simulink model "CANcommunicationmodule"  (R2024a)
settings: Solver=VariableStepAuto  StartTime=0.0  StopTime=10.0  RelTol=1e-3
undefined symbols (not defined in the file or in its folder): canChannel
libraries: canlib x4, canmsglib x3
settings Model: DataDictionary=BMS_System_dict1.sldd  Creator=hirah  LastModifiedBy=hirah

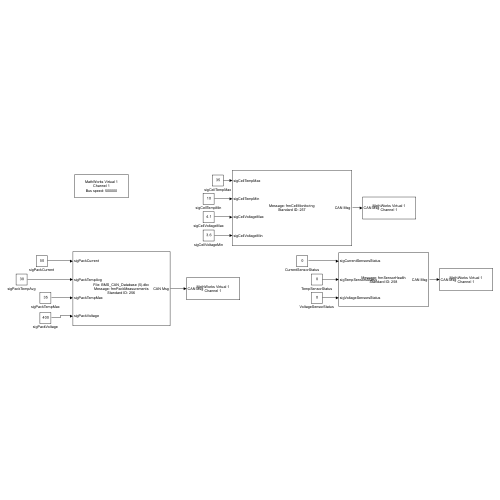
[thumbnail: Simulink's stored preview of the top-level diagram]
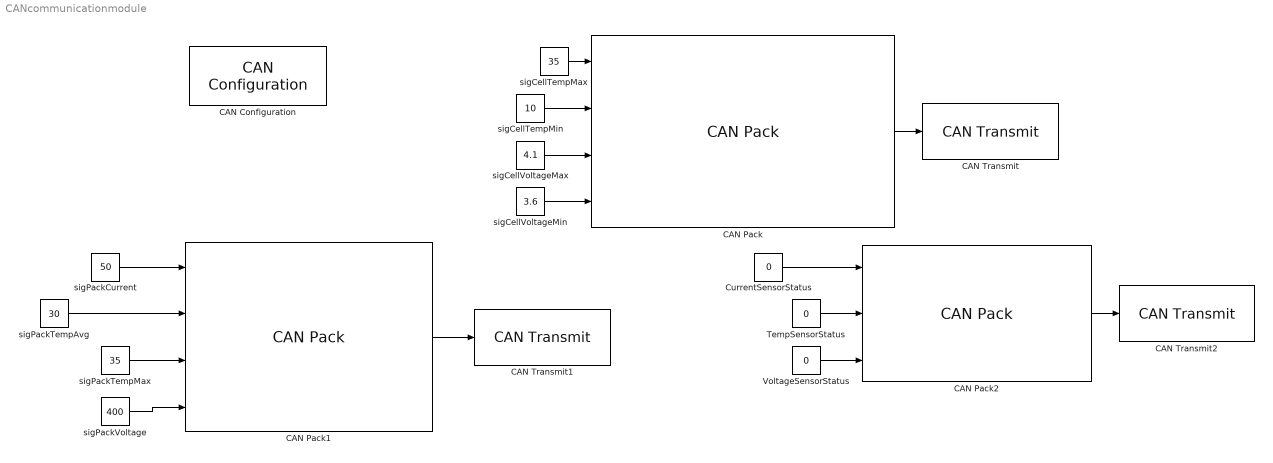
== system CANcommunicationmodule ==
  CAN Configuration : canlib/CAN Configuration  BlockHandle=788.0009  Device=MathWorks Virtual 1 (Channel 1)  DeviceMenu=MathWorks Virtual 1 (Channel 1)  ObjConstructor=canChannel('MathWorks', 'Virtual 1', 1)  BusSpeed=500000  EnableBitParameters=off  AckMode=Normal
  CAN Pack : canmsglib/CAN Pack  CANdbFile=C:\Users\hirah\Downloads\BMS_CAN_Database (5).dbc  MsgList=frmCellMonitoring  MsgName=frmCellMonitoring  MsgIDType=Standard (11-bit identifier)  MsgIdentifier=257  MsgLength=6  Remote=off  ApplyMinMax=off  BusOutput=off  SignalInfo={ 'sigCellTempMax', '32', '8', 'LE', 'unsigned', 'Standard', '0', '1', '-40', '-40', '150'; 'sigCellTempMin', '40', '8', 'LE', 'unsigned', 'Standard', '0', '1', '-40', '-40', '150'; 'sigCellVoltageMax', '0', '16', 'LE', 'unsigned', 'Standard', '0', '0.001', '0', '0', '5'; 'sigCellVoltageMin', '16', '16', 'LE', 'unsigned', 'Standard', '0', '0.001', '0', '0', '5' }
      settings: LibrarySourceBlock=canlib/CAN Pack  DataFormat=manually specified signals
  CAN Pack1 : canmsglib/CAN Pack  CANdbFile=C:\Users\hirah\Downloads\BMS_CAN_Database (5).dbc  MsgList=frmPackMeasurements  MsgName=frmPackMeasurements  MsgIDType=Standard (11-bit identifier)  MsgIdentifier=256  MsgLength=6  Remote=off  ApplyMinMax=off  BusOutput=off  SignalInfo={'sigPackCurrent','16','16','LE','signed','Standard','0','0.1','0','-400','400';'sigPackTempAvg','32','8','LE','unsigned','Standard','0','1','-40','-40','150';'sigPackTempMax','40','8','LE','unsigned','Standard','0','1','-40','-40','150';'sigPackVoltage','0','16','LE','unsigned','Standard','0','0.1','0','0','1000'}
      settings: LibrarySourceBlock=canlib/CAN Pack  DataFormat=CANdb specified signals
  CAN Pack2 : canmsglib/CAN Pack  CANdbFile=C:\Users\hirah\Downloads\BMS_CAN_Database (5).dbc  MsgList=frmSensorHealth  MsgName=frmSensorHealth  MsgIDType=Standard (11-bit identifier)  MsgIdentifier=258  MsgLength=3  Remote=off  ApplyMinMax=off  BusOutput=off  SignalInfo={ 'sigCurrentSensorsStatus', '8', '8', 'LE', 'unsigned', 'Standard', '0', '1', '0', '0', '3'; 'sigTempSensorsStatus', '16', '8', 'LE', 'unsigned', 'Standard', '0', '1', '0', '0', '3'; 'sigVoltageSensorsStatus', '0', '8', 'LE', 'unsigned', 'Standard', '0', '1', '0', '0', '3' }
      settings: LibrarySourceBlock=canlib/CAN Pack  DataFormat=manually specified signals
  CAN Transmit : canlib/CAN Transmit  BlockHandle=806.0001  Device=MathWorks Virtual 1 (Channel 1)  DeviceMenu=MathWorks Virtual 1 (Channel 1)  ObjConstructor=canChannel('MathWorks', 'Virtual 1', 1)  EnableEventTransmit=off  EnablePeriodicTransmit=off  MessagePeriod=1.000
  CAN Transmit1 : canlib/CAN Transmit  BlockHandle=808.0001  Device=MathWorks Virtual 1 (Channel 1)  DeviceMenu=MathWorks Virtual 1 (Channel 1)  ObjConstructor=canChannel('MathWorks', 'Virtual 1', 1)  EnableEventTransmit=off  EnablePeriodicTransmit=off  MessagePeriod=1.000
  CAN Transmit2 : canlib/CAN Transmit  BlockHandle=810.0001  Device=MathWorks Virtual 1 (Channel 1)  DeviceMenu=MathWorks Virtual 1 (Channel 1)  ObjConstructor=canChannel('MathWorks', 'Virtual 1', 1)  EnableEventTransmit=off  EnablePeriodicTransmit=off  MessagePeriod=1.000
  CurrentSensorStatus : Constant  Value=0  OutDataTypeStr=uint8
  TempSensorStatus : Constant  Value=0  OutDataTypeStr=uint8
  VoltageSensorStatus : Constant  Value=0  OutDataTypeStr=uint8
  sigCellTempMax : Constant  Value=35  OutDataTypeStr=int8
  sigCellTempMin : Constant  Value=10  OutDataTypeStr=int8
  sigCellVoltageMax : Constant  Value=4.1  OutDataTypeStr=double
  sigCellVoltageMin : Constant  Value=3.6  OutDataTypeStr=double
  sigPackCurrent : Constant  Value=50  OutDataTypeStr=double
  sigPackTempAvg : Constant  Value=30  OutDataTypeStr=double
  sigPackTempMax : Constant  Value=35  OutDataTypeStr=double
  sigPackVoltage : Constant  Value=400  OutDataTypeStr=double
  wires:
  sigCellTempMax/1 -> CAN Pack/1
  sigCellTempMin/1 -> CAN Pack/2
  sigCellVoltageMax/1 -> CAN Pack/3
  sigCellVoltageMin/1 -> CAN Pack/4
  CAN Pack/1 -> CAN Transmit/1
  sigPackCurrent/1 -> CAN Pack1/1
  sigPackTempAvg/1 -> CAN Pack1/2
  sigPackTempMax/1 -> CAN Pack1/3
  sigPackVoltage/1 -> CAN Pack1/4
  CAN Pack1/1 -> CAN Transmit1/1
  CAN Pack2/1 -> CAN Transmit2/1
  CurrentSensorStatus/1 -> CAN Pack2/1
  TempSensorStatus/1 -> CAN Pack2/2
  VoltageSensorStatus/1 -> CAN Pack2/3
